simulink model "Main_Model"  (R2022b)
settings: Solver=VariableStepAuto  StartTime=0.0  StopTime=2  FixedStep=1e-4  RelTol=1e-6
InitFcn:
  | Lfg=1.75e-3;
  | Lfc=3.5e-3;
  | Lf = Lfg +Lfc;
  | Cf=20e-6;
  | 
  | Lg=0.0035;
  | L=Lf+Lg;
  | Rg=0.5498*2;
  | k=0.707;
  | omega0 = 100*pi;
  | kp1=10;
  | ki1=250;
  | %kp1=10;
  | %ki1=250;
  | kp2=10;
  | ki2=250;
undefined symbols (not defined in the file): den_Tn2p_11, den_Tn2p_12, den_Tp2n_11, den_Tp2n_12, num_Tn2p_11, num_Tn2p_12, num_Tp2n_11, num_Tp2n_12
libraries: spsSeriesRLCBranchLib x12, slpidlib x9, spsControlledVoltageSourceLib x6, spsThreePhaseVIMeasurementLib x3, spsAlphaBetaZerotoabcLib x2, simulink x2, spsGroundLib x1, spspowerguiLib x1
(part 1 of 2)
settings Model: Creator=Sweet_J  LastModifiedBy=Sweet_J
settings DataIOCC: ReturnWorkspaceOutputs=off

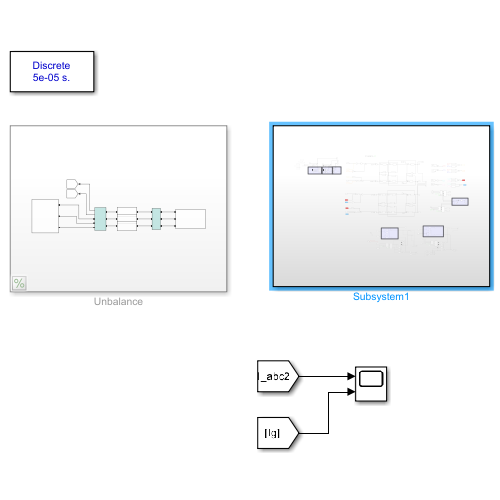
[thumbnail: Simulink's stored preview of the top-level diagram]
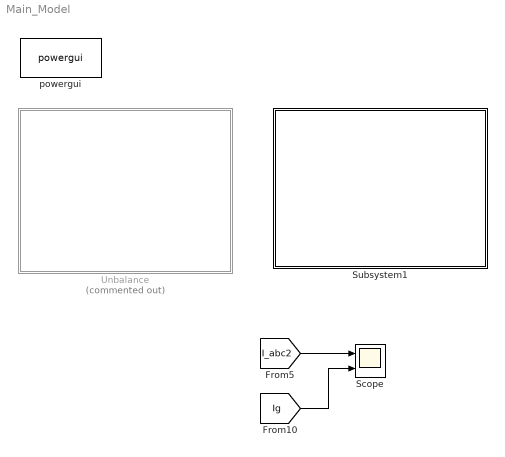
== system Main_Model ==
  Scope : Scope  NumInputPorts=2
  Subsystem1 : Subsystem
  Unbalance : Subsystem  Commented=on
  powergui : spspowerguiLib/powergui  Priority=1  SimulationMode=Discrete  SampleTime=5e-5  frequency=60  Iterations=50  frequencyindice=0  Pbase=100e6  ErrMax=1e-4  UnitsV=kV  UnitsW=MW  buscounter=0  FunctionMessages=off  echomessages=off  EnableUseOfTLC=off  CurrentSourceSwitches=off  DisableSnubberDevices=off  DisableRonSwitches=off  DisableVfSwitches=off  DisplayEquations=off  AutomaticDiscreteSolvers=off  SolverType=Tustin/Backward Euler (TBE)  Interpol=off  ExternalGateDelay=off  methode=off  Ts=100  x0status=blocks  SPID=on  SwTol=0  HookPort=off  NonlinearTolerance=1e-4  nMaxIteration=100  ContinueOnMaxIteration=off  RestoreLinks=warning  ResistiveCurrentMeasurement=off  Frange=[0:2:500]  Ylog=off  Xlog=on  ShowGrid=off  save=off  variable=ZData  structure=0  ZoomFFT=off  StartTime=0.0  cycles=1  DisplayStyle=1  fundamental=60  FreqAxis=off  MaxFrequency=1000  frequencyindicesteady=1  RmsSteady=1  display=off
  wires:
  [I_abc2] -> Scope/1
  [Ig] -> Scope/2

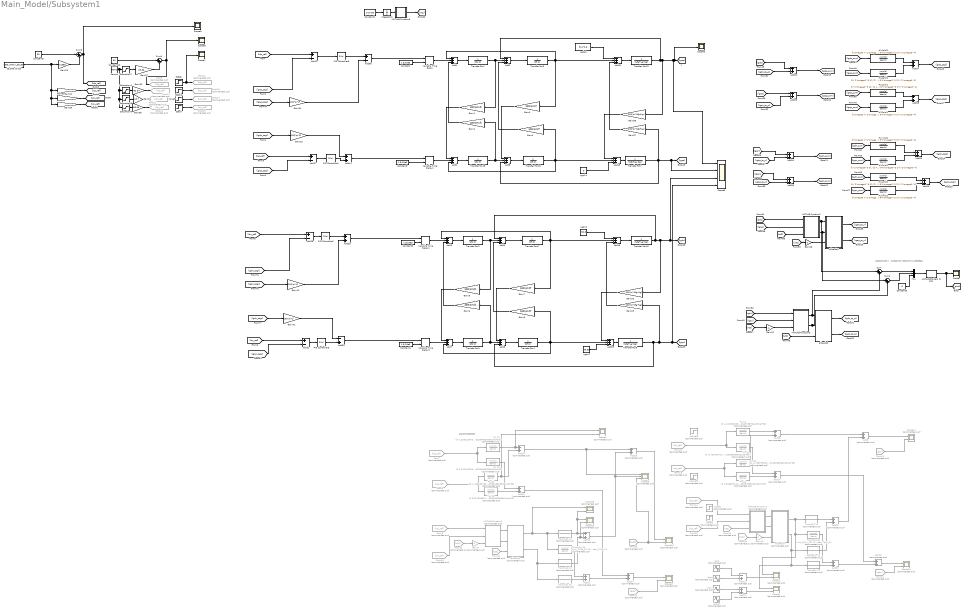
== system Main_Model/Subsystem1 ==
  note: 验证所求传函矩阵
  note: 这里其实说明了，系统真正的三相电流可以从哪里看出
  Add1 : Sum  Inputs=-++
  Add{9..10,12,14..15,17..18,20..23,25,27} (13 alike) : Sum  Commented=on
  Add11 : Sum  Commented=on  Inputs=-+
  Add2 : Sum  Inputs=-++
  Add24 : Sum  Inputs=-++
  Add{26,32..35,37..40,44} (10 alike) : Sum
  Add{28,31,36,42,47} (5 alike) : Sum  Inputs=+-
  Add29 : Sum  Inputs=++-
  Add{3..6,43,45} (6 alike) : Sum  Inputs=-+-
  Add30 : Sum  Inputs=-+
  Add7 : Sum  Inputs=++-
  Add8 : Sum  Inputs=++-
  Alpha-Beta-Zero to abc : spsAlphaBetaZerotoabcLib/Alpha-Beta-Zero to abc
      settings: LibrarySourceBlock=|
      | sps_lib/Control/Alpha-Beta-Zero
      | to abc
  Constant{,2..4} (4 alike) : Constant  Value=1.5/10e3
  Constant1 : Constant  Value=2*pi*50
  Constant10 : Constant  Value=50
  Constant5 : Constant  Value=0
  Constant9 : Constant  Value=50
  From10 : From  Commented=on  GotoTag=iqn_ref
  From{11..12,18..19} (4 alike) : From  Commented=on  GotoTag=wt2
  From13 : From  Commented=on  GotoTag=iqn_ref
  From14 : From  Commented=on  GotoTag=idp_ref
  From15 : From  Commented=on  GotoTag=iqp_ref
  From16 : From  Commented=on  GotoTag=igdp
  From17 : From  Commented=on  GotoTag=igqp
  From20 : From  Commented=on  GotoTag=igdn
  From21 : From  Commented=on  GotoTag=igqn
  From22 : From  Commented=on  GotoTag=idn_ref
  From7 : From  Commented=on  GotoTag=idp_ref
  From8 : From  Commented=on  GotoTag=iqp_ref
  From9 : From  Commented=on  GotoTag=idn_ref
  Gain{1..2,5..6} (4 alike) : Gain  Gain=100*pi*Lfc
  Gain10 : Gain  Commented=on  Gain=-1
  Gain22 : Gain  Gain=-1
  Gain{23,34,41..42} (4 alike) : Gain  Gain=100*pi*Lf
  Gain{25..26,37..38} (4 alike) : Gain  Gain=100*pi*(Lfg+Lg)
  Gain27 : Gain  Gain=25.56
  Gain28 : Gain  Gain=-1
  Gain29 : Gain  Gain=0.2556
  Gain{3..4,7..8} (4 alike) : Gain  Gain=100*pi*Cf
  Gain30 : Gain  Gain=-52.34
  Gain31 : Gain  Gain=-15.7
  Gain32 : Gain  Gain=-0.5234
  Gain33 : Gain  Gain=-0.157
  Gain35 : Gain  Gain=-0.5556
  Gain36 : Gain  Gain=-55.56
  Gain9 : Gain  Commented=on  Gain=-1
  Goto10 : Goto  Commented=on  GotoTag=iqp_ref
  Goto11 : Goto  Commented=on  GotoTag=idp_ref
  Goto12 : Goto  Commented=on  GotoTag=idn_ref
  Goto13 : Goto  Commented=on  GotoTag=iqp_ref
  Goto14 : Goto  Commented=on  GotoTag=idn_ref
  Goto15 : Goto  Commented=on  GotoTag=iqn_ref
  Goto16 : Goto  Commented=on  GotoTag=iqn_ref
  Goto9 : Goto  Commented=on  GotoTag=idp_ref
  H11n(s)2 : TransferFcn  Numerator=[k*omega0 k^2*omega0^2 4*k*omega0^3 2*k^2*omega0^4]  Denominator=[2 4*k*omega0 (2*k^2*omega0^2+8*omega0^2) 8*k*omega0^3 2*k^2*omega0^4]
  H11p(s)2 : TransferFcn  Numerator=[k*omega0 k^2*omega0^2 4*k*omega0^3 2*k^2*omega0^4]  Denominator=[2 4*k*omega0 (2*k^2*omega0^2+8*omega0^2) 8*k*omega0^3 2*k^2*omega0^4]
  H12n(s)2 : TransferFcn  Numerator=[k^2*omega0^3 0]  Denominator=[2 4*k*omega0 (2*k^2*omega0^2+8*omega0^2) 8*k*omega0^3 2*k^2*omega0^4]
  H12p(s)2 : TransferFcn  Numerator=[-k^2*omega0^3 0]  Denominator=[2 4*k*omega0 (2*k^2*omega0^2+8*omega0^2) 8*k*omega0^3 2*k^2*omega0^4]
  H21n(s)2 : TransferFcn  Numerator=[-k^2*omega0^3 0]  Denominator=[2 4*k*omega0 (2*k^2*omega0^2+8*omega0^2) 8*k*omega0^3 2*k^2*omega0^4]
  H21p(s)1 : TransferFcn  Numerator=[k^2*omega0^3 0]  Denominator=[2 4*k*omega0 (2*k^2*omega0^2+8*omega0^2) 8*k*omega0^3 2*k^2*omega0^4]
  H22n(s)2 : TransferFcn  Numerator=[k*omega0 k^2*omega0^2 4*k*omega0^3 2*k^2*omega0^4]  Denominator=[2 4*k*omega0 (2*k^2*omega0^2+8*omega0^2) 8*k*omega0^3 2*k^2*omega0^4]
  H22p(s)1 : TransferFcn  Numerator=[k*omega0 k^2*omega0^2 4*k*omega0^3 2*k^2*omega0^4]  Denominator=[2 4*k*omega0 (2*k^2*omega0^2+8*omega0^2) 8*k*omega0^3 2*k^2*omega0^4]
  Igdnref2 : Step  Commented=on  Time=0.5  After=-15.7  SampleTime=0
  Igqnref2 : Step  Commented=on  Time=0.5  After=-55.56  SampleTime=0
  Integrator1 : Integrator
  MATLAB Function1 : MATLAB Function  Commented=on  TreatAsAtomicUnit=on
  MATLAB Function2 : MATLAB Function  TreatAsAtomicUnit=on
  MATLAB Function3 : MATLAB Function  TreatAsAtomicUnit=on
  MATLAB Function4 : MATLAB Function  Commented=on  TreatAsAtomicUnit=on
  MATLAB Function5 : MATLAB Function  TreatAsAtomicUnit=on
  Mux : Mux  Inputs=3
  PID Controller{1..3,8} (4 alike) : slpidlib/PID Controller  Controller=PI  Form=Parallel  TimeDomain=Continuous-time  UseExternalTs=off  SampleTime=-1  IntegratorMethod=Forward Euler  FilterMethod=Forward Euler  ControllerParametersSource=internal  P=kp2  I=ki2  UseKiTs=off  D=0  N=100  UseFilter=on  TunerSelectOption=Transfer Function Based (PID Tuner App)  InitialConditionSource=internal  InitialConditionForIntegrator=0  InitialConditionForFilter=0  DifferentiatorICPrevScaledInput=0  ExternalReset=none  TrackingMode=off  Kt=1  LimitOutput=off  SatLimitsSource=internal  UpperSaturationLimit=5  LowerSaturationLimit=-5  LinearizeAsGain=on  AntiWindupMode=none  Kb=1  LimitIntegrator=off  UpperIntegratorSaturationLimit=inf  LowerIntegratorSaturationLimit=-inf  POutMin=[]  POutMax=[]  IOutMin=[]  IOutMax=[]  DOutMin=[]  DOutMax=[]  NOutMin=[]  NOutMax=[]  SumOutMin=[]  SumOutMax=[]  SaturationOutMin=[]  SaturationOutMax=[]  PParamMin=[]  PParamMax=[]  IParamMin=[]  IParamMax=[]  DParamMin=[]  DParamMax=[]  NParamMin=[]  NParamMax=[]  KbParamMin=[]  KbParamMax=[]  KtParamMin=[]  KtParamMax=[]  KbOutMin=[]  KbOutMax=[]  KtOutMin=[]  KtOutMax=[]  IntegratorOutMin=[]  IntegratorOutMax=[]  FilterOutMin=[]  FilterOutMax=[]  SumI1OutMin=[]  SumI1OutMax=[]  SumI2OutMin=[]  SumI2OutMax=[]  SumI3OutMin=[]  SumI3OutMax=[]  SumI4OutMin=[]  SumI4OutMax=[]  SumDOutMin=[]  SumDOutMax=[]  DifferentiatorOutMin=[]  DifferentiatorOutMax=[]  FilterDiffOutCoefMin=[]  FilterDiffOutCoefMax=[]  ReciprocalOutMin=[]  ReciprocalOutMax=[]  SumDenOutMin=[]  SumDenOutMax=[]  SumNumOutMin=[]  SumNumOutMax=[]  DivideOutMin=[]  DivideOutMax=[]  UdiffTsProdOutMin=[]  UdiffTsProdOutMax=[]  NTsProdOutMin=[]  NTsProdOutMax=[]  UintegralTsProdOutMin=[]  UintegralTsProdOutMax=[]  UngainTsProdOutMin=[]  UngainTsProdOutMax=[]  ClampingZeroOutDataTypeStr=Inherit: Inherit via back propagation  ClampingZeroOutMin=[]  ClampingZeroOutMax=[]  FilterDenConstantOutDataTypeStr=Inherit: Inherit via back propagation  FilterDenConstantOutMin=[]  FilterDenConstantOutMax=[]  PCopyOutDataTypeStr=Inherit: Inherit via back propagation  PCopyOutMin=[]  PCopyOutMax=[]  NCopyOutDataTypeStr=Inherit: Inherit via back propagation  NCopyOutMin=[]  NCopyOutMax=[]  IntegratorContinuousStateAttributes=''  IntegratorStateMustResolveToSignalObject=off  IntegratorRTWStateStorageClass=Auto  FilterContinuousStateAttributes=''  FilterStateMustResolveToSignalObject=off  FilterRTWStateStorageClass=Auto  ParallelPVariant=InternalParameters  IdealPVariant=Disabled  IVariant=InternalParameters  DVariant=Disabled  IntegratorVariant=Continuous  SatVariant=Disabled  AWVariant=Passthrough  PCopyVariant=Disabled  TRVariant=Disabled  FdbkBlocksVariant=Forward  IdealPFdbkVariant=Disabled  SatFdbkVariant=Disabled  DerivativeFilterVariant=Disabled  NVariant=Disabled  NCopyVariant=Disabled_SignalSpec  FilterICVariant=Disabled  IntegratorICVariant=InternalICs  ExternalResetVariant=Disabled  TRSumVariant=Passthrough  SumFdbkVariant=Disabled  SumVariant=Sum_PI  TsampFilterVariant=InternalTs  TsampNgainVariant=Passthrough  TsampIntegralVariant=Passthrough  ExternalSaturationOutDataTypeStr=Inherit: Same as second input
  Ramp4 : simulink/Sources/Ramp  slope=1/0.05  start=0.5  InitialOutput=0
  S5_500-优化值 : FromWorkspace  VariableName=data_matrix_S5_500  SampleTime=1e-4  OutputAfterFinalValue=Holding final value
  Saturation{4..7} (4 alike) : Saturate  UpperLimit=1
  Scope{,5..7,9} (5 alike) : Scope
  Scope{1..2,4,10..14,16} (9 alike) : Scope  Commented=on  NumInputPorts=2
  Scope3 : Scope  NumInputPorts=4
  Scope8 : Scope  Commented=on  NumInputPorts=3
  Step7 : Step  Time=0.5  After=-55.56  SampleTime=0
  Sum : Sum  Inputs=|++
  Sum1 : Sum  Inputs=|++
  Sum5 : Sum  Inputs=|+-
  Sum6 : Sum  Inputs=|+-
  Tn_11 : TransferFcn  Commented=on  Numerator="[0\t-1.01989600835735e-05\t-1.17900641885587\t27210822483.3065\t2.20664229038769e+15\t6.24118002886548e+19\t2.23888969085823e+23\t-1.87897168317480e+28\t-1.72747667412133e+31\t1.49299225089427e+37\t3.46754860086783e+41\t3.72395139767584e+45\t2.75969527472527e+49\t2.13218589100970e+53\t7.75699540504486e+56\t4.72648195947321e+60\t8.87634219530409e+63\t3.90830665381887e+67\t3.37200315132574e+70\t5.07472961316367e+73\t2.90981583243429e+76\t2.03203948734923e+79\t7.99056387196165e+81\t2.55933616110458e+84\t5.67621915091599e+86\t8.56295738691479e+88\t1.11882265410070e+91\t4.19269885253059e+92\t4.62854501341626e+93\t1.05501449453161e+90]"  Denominator="[1\t161278.621717248\t12035279516.7795\t542695985224921\t1.63257064864896e+19\t3.43390119397054e+23\t5.20049258153112e+27\t5.86772441336057e+31\t5.22760881524642e+35\t3.91267714232162e+39\t2.45413237239549e+43\t1.26235138927125e+47\t6.03726802536307e+50\t2.07018153285052e+54\t7.71850484834772e+57\t1.60031377689575e+61\t4.41534429030222e+64\t4.42330190486357e+67\t6.10017406906532e+70\t3.90204803066969e+73\t3.02442391656399e+76\t1.31463112199984e+79\t6.03213029135759e+81\t1.66887439356409e+84\t4.66750897142887e+86\t7.17549900075772e+88\t1.10373386868736e+91\t4.20898521075049e+92\t4.62821769543011e+93\t-2.01082889062291e+90]"
  Tn_12 : TransferFcn  Commented=on  Numerator="[0\t-4.73887980077529e-07\t-0.118436122586675\t-9193.30022294537\t-25646023787018.2\t-2.07793020544197e+18\t-5.82766629864322e+22\t-1.74505672449969e+26\t1.86276154721117e+31\t1.74470630730339e+34\t-1.43701084661191e+40\t-3.26090058003804e+44\t-3.26037804347025e+48\t-2.06927357042730e+52\t-1.50382199874050e+56\t-4.36162665974338e+59\t-2.45036259999236e+63\t-3.47377720397907e+66\t-1.31801840386399e+70\t-9.21889552517163e+72\t-1.38149069182804e+76\t-6.51712223024236e+78\t-4.53944031524944e+81\t-1.44387747033367e+84\t-3.90301534160538e+86\t-5.52809852598918e+88\t-2.66091379078351e+90\t-3.75543559155808e+91\t-1.49408154389136e+89\t-7.00886380960308e+89]"  Denominator="[1\t161278.621717248\t12035279516.7795\t542695985224921\t1.63257064864896e+19\t3.43390119397054e+23\t5.20049258153112e+27\t5.86772441336057e+31\t5.22760881524642e+35\t3.91267714232162e+39\t2.45413237239549e+43\t1.26235138927125e+47\t6.03726802536307e+50\t2.07018153285052e+54\t7.71850484834772e+57\t1.60031377689575e+61\t4.41534429030222e+64\t4.42330190486357e+67\t6.10017406906532e+70\t3.90204803066969e+73\t3.02442391656399e+76\t1.31463112199984e+79\t6.03213029135759e+81\t1.66887439356409e+84\t4.66750897142887e+86\t7.17549900075772e+88\t1.10373386868736e+91\t4.20898521075049e+92\t4.62821769543011e+93\t-2.01082889062291e+90]"
  Tn_21 : TransferFcn  Commented=on  Numerator="[0\t-2.72575672494487e-05\t-2.67780697081252\t-114599.451612093\t25642942591020.4\t2.07787868086678e+18\t5.82758566377686e+22\t1.74491674822968e+26\t-1.86277964459509e+31\t-1.74482881481782e+34\t1.43701045799572e+40\t3.26090034418790e+44\t3.26037826604666e+48\t2.06927358937222e+52\t1.50382192123535e+56\t4.36162780809189e+59\t2.45036177516416e+63\t3.47378233210236e+66\t1.31801708965542e+70\t9.21896059568848e+72\t1.38148936783182e+76\t6.51716065391267e+78\t4.53943833205246e+81\t1.44387765769510e+84\t3.90311991195425e+86\t5.52841692189602e+88\t2.66100296918848e+90\t3.75453399799371e+91\t-1.15709472803773e+89\t-4.22449198140034e+88]"  Denominator="[1\t161278.621717248\t12035279516.7795\t542695985224921\t1.63257064864896e+19\t3.43390119397054e+23\t5.20049258153112e+27\t5.86772441336057e+31\t5.22760881524642e+35\t3.91267714232162e+39\t2.45413237239549e+43\t1.26235138927125e+47\t6.03726802536307e+50\t2.07018153285052e+54\t7.71850484834772e+57\t1.60031377689575e+61\t4.41534429030222e+64\t4.42330190486357e+67\t6.10017406906532e+70\t3.90204803066969e+73\t3.02442391656399e+76\t1.31463112199984e+79\t6.03213029135759e+81\t1.66887439356409e+84\t4.66750897142887e+86\t7.17549900075772e+88\t1.10373386868736e+91\t4.20898521075049e+92\t4.62821769543011e+93\t-2.01082889062291e+90]"
  Tn_22 : TransferFcn  Commented=on  Numerator="[0\t3.66865324272166e-06\t-0.371826229889401\t27210820197.5691\t2.20664078258463e+15\t6.24117473554497e+19\t2.23888231391279e+23\t-1.87897185981957e+28\t-1.72747197520496e+31\t1.49299226921904e+37\t3.46754859641349e+41\t3.72395142079573e+45\t2.75969522576048e+49\t2.13218587839097e+53\t7.75699545713972e+56\t4.72648184009947e+60\t8.87634279451460e+63\t3.90830630184088e+67\t3.37200348967812e+70\t5.07472544820159e+73\t2.90981176456342e+76\t2.03203651448596e+79\t7.99054716401335e+81\t2.55934516074338e+84\t5.67629559985087e+86\t8.56289570963446e+88\t1.11878390677472e+91\t4.19253851985844e+92\t4.62825157508569e+93\t-2.00117520670361e+90]"  Denominator="[1\t161278.621717248\t12035279516.7795\t542695985224921\t1.63257064864896e+19\t3.43390119397054e+23\t5.20049258153112e+27\t5.86772441336057e+31\t5.22760881524642e+35\t3.91267714232162e+39\t2.45413237239549e+43\t1.26235138927125e+47\t6.03726802536307e+50\t2.07018153285052e+54\t7.71850484834772e+57\t1.60031377689575e+61\t4.41534429030222e+64\t4.42330190486357e+67\t6.10017406906532e+70\t3.90204803066969e+73\t3.02442391656399e+76\t1.31463112199984e+79\t6.03213029135759e+81\t1.66887439356409e+84\t4.66750897142887e+86\t7.17549900075772e+88\t1.10373386868736e+91\t4.20898521075049e+92\t4.62821769543011e+93\t-2.01082889062291e+90]"
  Tp_11 : TransferFcn  Commented=on  Numerator="[0\t-1.25322284335350e-05\t-2.02740537788495\t27210737835.9859\t2.20663793840066e+15\t6.24116626296036e+19\t2.23886077261772e+23\t-1.87897588898611e+28\t-1.72752135679541e+31\t1.49299184770071e+37\t3.46754821681792e+41\t3.72395106130426e+45\t2.75969508892492e+49\t2.13218578823217e+53\t7.75699430851545e+56\t4.72648172209308e+60\t8.87633831828796e+63\t3.90830600643315e+67\t3.37199825873036e+70\t5.07472177909344e+73\t2.90980757242417e+76\t2.03202861702974e+79\t7.99052798454746e+81\t2.55932291602922e+84\t5.67622759908534e+86\t8.56290284779787e+88\t1.11878404420830e+91\t4.19254404340210e+92\t4.62834852627690e+93]"  Denominator="[1\t161278.621529395\t12035279456.2977\t542695979191906\t1.63257061733538e+19\t3.43390109552110e+23\t5.20049238260333e+27\t5.86772414805569e+31\t5.22760856883647e+35\t3.91267695209602e+39\t2.45413222504702e+43\t1.26235129378665e+47\t6.03726748464878e+50\t2.07018118935140e+54\t7.71850362457027e+57\t1.60031311177394e+61\t4.41534276008939e+64\t4.42329659655974e+67\t6.10016546580316e+70\t3.90203985540913e+73\t3.02441198394233e+76\t1.31462548198536e+79\t6.03210232716645e+81\t1.66887043911015e+84\t4.66748787692584e+86\t7.17548130205310e+88\t1.10372137417744e+91\t4.20897950841205e+92\t4.62834862809614e+93]"
  Tp_12 : TransferFcn  Commented=on  Numerator="[0\t-1.18608236314470e-05\t-1.75109677806806\t-114697.716307309\t25641287601788.2\t2.07781430026798e+18\t5.82747088748898e+22\t1.74480497060541e+26\t-1.86278961312241e+31\t-1.74496642291660e+34\t1.43700919800844e+40\t3.26089973839346e+44\t3.26037735424563e+48\t2.06927349019002e+52\t1.50382186060258e+56\t4.36162596446295e+59\t2.45036239722728e+63\t3.47377484676323e+66\t1.31801807759520e+70\t9.21888581644634e+72\t1.38148983839453e+76\t6.51708864184348e+78\t4.53943011483970e+81\t1.44387260922491e+84\t3.90302852492583e+86\t5.52817130126409e+88\t2.66083943958935e+90\t3.75471287071865e+91\t-1.93887588410211e+87]"  Denominator="[1\t161278.621529395\t12035279456.2977\t542695979191906\t1.63257061733538e+19\t3.43390109552110e+23\t5.20049238260333e+27\t5.86772414805569e+31\t5.22760856883647e+35\t3.91267695209602e+39\t2.45413222504702e+43\t1.26235129378665e+47\t6.03726748464878e+50\t2.07018118935140e+54\t7.71850362457027e+57\t1.60031311177394e+61\t4.41534276008939e+64\t4.42329659655974e+67\t6.10016546580316e+70\t3.90203985540913e+73\t3.02441198394233e+76\t1.31462548198536e+79\t6.03210232716645e+81\t1.66887043911015e+84\t4.66748787692584e+86\t7.17548130205310e+88\t1.10372137417744e+91\t4.20897950841205e+92\t4.62834862809614e+93]"
  Tp_21 : TransferFcn  Commented=on  Numerator="[0\t2.94216760674153e-05\t4.42093407247836\t300641.920787539\t-25633527507541.4\t-2.07759953751829e+18\t-5.82705540457892e+22\t-1.74422205010133e+26\t1.86285087700518e+31\t1.74546015222327e+34\t-1.43700600599724e+40\t-3.26089770519802e+44\t-3.26037591493240e+48\t-2.06927290231164e+52\t-1.50382156142686e+56\t-4.36162560590497e+59\t-2.45036234473766e+63\t-3.47377754442195e+66\t-1.31801819198073e+70\t-9.21892944521939e+72\t-1.38148590156662e+76\t-6.51711111353095e+78\t-4.53942941502323e+81\t-1.44387357287478e+84\t-3.90304696099191e+86\t-5.52822127622576e+88\t-2.66087906457575e+90\t-3.75479198654529e+91\t3.61407592855685e+86]"  Denominator="[1\t161278.621529395\t12035279456.2977\t542695979191906\t1.63257061733538e+19\t3.43390109552110e+23\t5.20049238260333e+27\t5.86772414805569e+31\t5.22760856883647e+35\t3.91267695209602e+39\t2.45413222504702e+43\t1.26235129378665e+47\t6.03726748464878e+50\t2.07018118935140e+54\t7.71850362457027e+57\t1.60031311177394e+61\t4.41534276008939e+64\t4.42329659655974e+67\t6.10016546580316e+70\t3.90203985540913e+73\t3.02441198394233e+76\t1.31462548198536e+79\t6.03210232716645e+81\t1.66887043911015e+84\t4.66748787692584e+86\t7.17548130205310e+88\t1.10372137417744e+91\t4.20897950841205e+92\t4.62834862809614e+93]"
  Tp_22 : TransferFcn  Commented=on  Numerator="[0\t3.60780582170835e-06\t0.508903300575527\t27210914613.7454\t2.20664521469668e+15\t6.24118611598372e+19\t2.23889957097262e+23\t-1.87897006618828e+28\t-1.72745122527653e+31\t1.49299249961866e+37\t3.46754864365711e+41\t3.72395127329797e+45\t2.75969521169702e+49\t2.13218581722092e+53\t7.75699456142154e+56\t4.72648171699777e+60\t8.87633866859007e+63\t3.90830591483511e+67\t3.37199835513012e+70\t5.07472114504140e+73\t2.90980609802614e+76\t2.03203336431316e+79\t7.99052910989882e+81\t2.55933700246574e+84\t5.67627031006410e+86\t8.56293334609155e+88\t1.11878556056281e+91\t4.19254427849679e+92\t4.62834263680031e+93]"  Denominator="[1\t161278.621529395\t12035279456.2977\t542695979191906\t1.63257061733538e+19\t3.43390109552110e+23\t5.20049238260333e+27\t5.86772414805569e+31\t5.22760856883647e+35\t3.91267695209602e+39\t2.45413222504702e+43\t1.26235129378665e+47\t6.03726748464878e+50\t2.07018118935140e+54\t7.71850362457027e+57\t1.60031311177394e+61\t4.41534276008939e+64\t4.42329659655974e+67\t6.10016546580316e+70\t3.90203985540913e+73\t3.02441198394233e+76\t1.31462548198536e+79\t6.03210232716645e+81\t1.66887043911015e+84\t4.66748787692584e+86\t7.17548130205310e+88\t1.10372137417744e+91\t4.20897950841205e+92\t4.62834862809614e+93]"
  Transfer Fcn{1..3,18} (4 alike) : TransferFcn  Denominator=[Lfc 0]
  Transfer Fcn{7..8,13,16} (4 alike) : TransferFcn  Denominator=[(Lfg+Lg) Rg]
  Transfer Fcn{4..6,19} (4 alike) : TransferFcn  Denominator=[Cf 0]
  Tsumn2p_11 : TransferFcn  Commented=on  Numerator=num_Tn2p_11  Denominator=den_Tn2p_11
  Tsumn2p_12 : TransferFcn  Commented=on  Numerator=num_Tn2p_12  Denominator=den_Tn2p_12
  Tsumn2p_21 : TransferFcn  Commented=on  Numerator=num_Tn2p_12*(-1)  Denominator=den_Tn2p_12
  Tsumn2p_22 : TransferFcn  Commented=on  Numerator=num_Tn2p_11  Denominator=den_Tn2p_11
  Tsump2n_11 : TransferFcn  Commented=on  Numerator=num_Tp2n_11  Denominator=den_Tp2n_11
  Tsump2n_12 : TransferFcn  Commented=on  Numerator=num_Tp2n_12  Denominator=den_Tp2n_12
  Tsump2n_21 : TransferFcn  Commented=on  Numerator=num_Tp2n_12*(-1)  Denominator=den_Tp2n_11
  Tsump2n_22 : TransferFcn  Commented=on  Numerator=num_Tp2n_11  Denominator=den_Tp2n_11
  Variable Time Delay{,1..3} (4 alike) : VariableTransportDelay  MaximumDelay=10
  albe-dq1 : MATLAB Function  Commented=on  TreatAsAtomicUnit=on
  albe-dq2 : MATLAB Function  TreatAsAtomicUnit=on
  albe-dq3 : MATLAB Function  TreatAsAtomicUnit=on
  albe-dq4 : MATLAB Function  Commented=on  TreatAsAtomicUnit=on
  idcos : Sin  Commented=on  Amplitude=24.44  Frequency=2*2*50*pi  Phase=pi/2  SampleTime=0
  idnref : Step  Time=0.5  After=-15.7  SampleTime=0
  idpref1 : Step  Commented=on  Time=0.5  Before=50  After=24.44  SampleTime=0
  idsin1 : Sin  Commented=on  Amplitude=24.44  Frequency=2*2*50*pi  SampleTime=0
  iqcos1 : Sin  Commented=on  Amplitude=-52.34  Frequency=2*2*50*pi  Phase=pi/2  SampleTime=0
  iqpref1 : Step  Commented=on  Time=0.5  After=-52.34  SampleTime=0
  iqsin : Sin  Commented=on  Amplitude=-52.34  Frequency=2*2*50*pi  SampleTime=0
  ugdn2 : Constant  Value=80.8
  ugdp1 : Constant  Value=311*0.6
  ugq+4 : Constant  Value=0
  ugqn2 : Constant  Value=46.65
  转换后 : Step  Time=0.5  Before=50  After=24.44  SampleTime=0
  转换后2 : Step  Time=0.5  After=-52.34  SampleTime=0
  tag scope: I_abc2=global
  wires:
  [igqn] -> MATLAB Function3/2(uq)
  albe-dq2/1(vd) -> [igdn_to_p]
  [igdp] -> Add32/1
  Add33/1 -> [igqp_sum]
  [wt2] -> Gain22/1
  [igdn] -> MATLAB Function3/1(ud)
  [wt2] -> albe-dq2/3(ph)
  [wt2] -> Gain28/1
  Gain22/1 -> MATLAB Function3/3(ph)
  [igqp] -> Add33/1
  albe-dq3/2(vq) -> [igqp_to_n]
  albe-dq3/1(vd) -> [igdp_to_n]
  Integrator1/1 -> MATLAB Function5/1(u)
  [igqp_sum] -> H22p(s)1/1
  [igdn_to_p] -> Add32/2
  H11p(s)2/1 -> Add37/1
  [igdp] -> MATLAB Function2/1(ud)
  [wt2] -> MATLAB Function2/3(ph)
  MATLAB Function2/2(ub) -> Sum1/1, albe-dq3/2(vbeta)  "v_bn"
  [igqn_sum] -> H12n(s)2/1
  [igqp] -> MATLAB Function2/2(uq)
  MATLAB Function2/1(ua) -> albe-dq3/1(valpha), Sum/1  "v_an"
  Add34/1 -> [igdn_sum]
  Gain28/1 -> albe-dq3/3(ph)
  H22n(s)2/1 -> Add40/2
  [igqp_to_n] -> Add35/2
  [igqn] -> Add35/1
  [igdp_sum] -> H11p(s)2/1
  H12p(s)2/1 -> Add37/2
  Add37/1 -> [igdp_sogi]
  albe-dq2/2(vq) -> [igqn_to_p]
  [igdp_sum] -> H21p(s)1/1
  H22p(s)1/1 -> Add38/2
  H12n(s)2/1 -> Add39/2
  [igqn_sum] -> H22n(s)2/1
  Add40/1 -> [igqn_sogi]
  Add30/1 -> Variable Time Delay3/1  "usq"
  ugdn2/1 -> Add45/1
  [igdn_sogi] -> Gain41/1
  Add35/1 -> [igqn_sum]
  [igqn_sogi] -> Gain42/1
  [igqp_sogi] -> Add47/2
  Add43/1 -> Transfer Fcn7/1
  [igdp_sogi] -> Gain23/1
  Transfer Fcn7/1 -> Gain37/1, Add5/3, Scope3/2, [igqp]  "igq+"
  ugq+4/1 -> Add43/3
  Add42/1 -> PID Controller8/1
  Add29/1 -> Transfer Fcn8/1
  H11n(s)2/1 -> Add39/1
  ugdp1/1 -> Add24/1
  Add36/1 -> Variable Time Delay/1  "usd"
  H21n(s)2/1 -> Add40/1
  [igdn_sum] -> H11n(s)2/1
  [igqn_to_p] -> Add33/2
  Gain34/1 -> Add36/2
  [igdp_to_n] -> Add34/2
  Gain37/1 -> Add24/3
  [igdn] -> Add34/1
  Add24/1 -> Transfer Fcn13/1
  [igdp_sogi] -> Add42/2
  Add47/1 -> PID Controller1/1
  PID Controller3/1 -> Add30/2
  Gain23/1 -> Add44/1
  [igqp_sogi] -> Gain34/1
  PID Controller8/1 -> Add36/1
  MATLAB Function3/2(ub) -> Sum1/2, albe-dq2/2(vbeta)  "v_bn"
  H21p(s)1/1 -> Add38/1
  Add38/1 -> [igqp_sogi]
  PID Controller2/1 -> Add26/1
  MATLAB Function3/1(ua) -> Sum/2, albe-dq2/1(valpha)  "v_an"
  Add28/1 -> PID Controller2/1
  Gain42/1 -> Add26/2
  [igdn_sum] -> H21n(s)2/1
  ugqn2/1 -> Add29/3
  Gain26/1 -> Add29/1
  Add31/1 -> PID Controller3/1
  Add45/1 -> Transfer Fcn16/1
  Gain25/1 -> Add45/3
  Add32/1 -> [igdp_sum]
  Constant1/1 -> Integrator1/1
  Add44/1 -> Variable Time Delay1/1  "usq"
  PID Controller1/1 -> Add44/2
  Gain38/1 -> Add43/1
  [igdn_sogi] -> Add28/2
  Gain41/1 -> Add30/1
  [igqp_sum] -> H12p(s)2/1
  Transfer Fcn13/1 -> Add2/1, Gain38/1, Scope3/1, Scope6/1, [igdp]  "igd+"
  Add39/1 -> [igdn_sogi]
  Constant/1 -> Variable Time Delay/2
  Constant2/1 -> Variable Time Delay1/2
  Constant3/1 -> Variable Time Delay2/2
  Add26/1 -> Variable Time Delay2/1  "usq"
  Constant4/1 -> Variable Time Delay3/2
  Sum/1 -> Mux/1
  Sum1/1 -> Mux/2
  Constant5/1 -> Mux/3
  Mux/1 -> Alpha-Beta-Zero to abc/1
  Alpha-Beta-Zero to abc/1 -> [I_abc2], Scope/1
  MATLAB Function5/1(y) -> [wt2]
  Variable Time Delay/1 -> Add1/2
  Transfer Fcn1/1 -> Gain1/1, Add2/2  "i1d+"
  Add2/1 -> Transfer Fcn5/1
  Transfer Fcn5/1 -> Add24/2, Gain3/1, Add1/1  "vc+"
  Add1/1 -> Transfer Fcn1/1
  Gain1/1 -> Add4/1
  Gain2/1 -> Add1/3
  Add4/1 -> Transfer Fcn18/1
  Transfer Fcn19/1 -> Add4/3, Add43/2, Gain4/1  "vc+"
  Add5/1 -> Transfer Fcn19/1
  Transfer Fcn18/1 -> Gain2/1, Add5/2  "i1q+"
  Variable Time Delay1/1 -> Add4/2
  Gain3/1 -> Add5/1
  Gain4/1 -> Add2/3
  Gain8/1 -> Add6/3
  Gain7/1 -> Add8/1
  Transfer Fcn3/1 -> Add8/2, Gain6/1  "i1q-"
  Add8/1 -> Transfer Fcn4/1
  Transfer Fcn4/1 -> Add29/2, Gain8/1, Add7/3  "vc-"
  Add7/1 -> Transfer Fcn3/1
  Gain6/1 -> Add3/3
  Gain5/1 -> Add7/1
  Add3/1 -> Transfer Fcn2/1
  Transfer Fcn6/1 -> Gain7/1, Add45/2, Add3/1  "vc-"
  Add6/1 -> Transfer Fcn6/1
  Transfer Fcn2/1 -> Add6/2, Gain5/1  "i1d-"
  Transfer Fcn16/1 -> Add6/1, Gain26/1, Scope3/3, [igdn]  "igd-"
  Transfer Fcn8/1 -> Scope3/4, [igqn], Gain25/1, Add8/3  "igq-"
  Variable Time Delay2/1 -> Add3/2
  Variable Time Delay3/1 -> Add7/2
  [igqn_sogi] -> Add31/2
  From7/1 -> Tp_11/1, Tp_21/1
  From22/1 -> Tn_11/1, Tn_21/1
  Tn_11/1 -> Add18/1
  Tn_21/1 -> Add17/1
  Gain9/1 -> MATLAB Function1/3(ph)
  MATLAB Function1/2(ub) -> albe-dq1/2(vbeta)  "v_bn"
  From12/1 -> Gain9/1
  From11/1 -> albe-dq1/3(ph)
  MATLAB Function1/1(ua) -> albe-dq1/1(valpha)  "v_an"
  From9/1 -> MATLAB Function1/1(ud)
  From10/1 -> MATLAB Function1/2(uq)
  From13/1 -> Tn_12/1, Tn_22/1
  Tn_22/1 -> Add17/2
  Tn_12/1 -> Add18/2
  Add18/1 -> Add9/1
  albe-dq1/2(vq) -> Tsumn2p_22/1, Tsumn2p_12/1
  Tsumn2p_11/1 -> Scope14/1, Scope16/2, Add20/1
  Tsumn2p_12/1 -> Scope14/2, Add20/2
  Tsumn2p_22/1 -> Add21/2
  Tsumn2p_21/1 -> Add21/1
  Add25/1 -> Scope10/1  "idp_theory"
  From16/1 -> Scope8/3, Scope10/2  "idp_simulation"
  Add27/1 -> Scope11/1  "iqp_theory"
  From17/1 -> Scope11/2  "iqp_simulation"
  Tsump2n_21/1 -> Add23/1
  Tsump2n_22/1 -> Add23/2
  Tsump2n_12/1 -> Add22/2
  Tsump2n_11/1 -> Add22/1
  From18/1 -> Gain10/1
  MATLAB Function4/2(ub) -> albe-dq4/2(vbeta)  "v_bn"
  MATLAB Function4/1(ua) -> albe-dq4/1(valpha)  "v_an"
  albe-dq4/1(vd) -> Tsump2n_11/1, Scope1/1, Tsump2n_21/1
  albe-dq4/2(vq) -> Scope2/1, Tsump2n_22/1, Tsump2n_12/1
  Add22/1 -> Add9/2
  From20/1 -> Scope12/2  "idn_simulation"
  Add23/1 -> Add10/2
  From21/1 -> Scope13/2  "iqn_simulation"
  From8/1 -> Tp_12/1, Tp_22/1
  Tp_11/1 -> Scope4/1, Add14/1
  Tp_21/1 -> Add15/1
  Tp_22/1 -> Add15/2
  Add14/1 -> Scope8/1, Add25/1
  Add15/1 -> Add27/1
  Add20/1 -> Add25/2, Scope8/2
  Add21/1 -> Add27/2
  Add17/1 -> Add10/1
  Add10/1 -> Scope13/1  "iqn_theory"
  Add9/1 -> Scope12/1  "idn_theory"
  iqsin/1 -> Add11/1
  idcos/1 -> Add11/2
  iqcos1/1 -> Add12/2
  idsin1/1 -> Add12/1
  Add11/1 -> Scope1/2  "d"
  Add12/1 -> Scope2/2  "q"
  From14/1 -> MATLAB Function4/1(ud)
  From15/1 -> MATLAB Function4/2(uq)
  From19/1 -> MATLAB Function4/3(ph)
  Gain10/1 -> albe-dq4/3(ph)
  [idp_ref] -> Add42/1
  [iqp_ref] -> Add47/1
  [idn_ref] -> Add28/1
  [iqn_ref] -> Add31/1
  albe-dq1/1(vd) -> Scope16/1, Tsumn2p_11/1, Tsumn2p_21/1
  Gain31/1 -> Goto12/1  "idn_ref"
  Saturation4/1 -> Gain30/1  "斜坡"
  Constant9/1 -> Sum5/1
  Gain29/1 -> Sum5/2  "优化idp_ref"
  Gain30/1 -> Goto10/1
  Saturation5/1 -> Gain31/1
  Sum6/1 -> Scope5/1, Goto9/1
  Gain27/1 -> Sum6/2
  Ramp4/1 -> Saturation4/1, Saturation6/1, Saturation5/1, Saturation7/1
  Constant10/1 -> Sum6/1
  Gain32/1 -> [iqp_ref]  "iqp_ref"
  Gain33/1 -> [idn_ref]  "idn_ref"
  Sum5/1 -> [idp_ref], Scope9/1  "idp_ref"
  Gain36/1 -> Goto16/1
  Saturation7/1 -> Gain27/1  "斜坡"
  Gain35/1 -> [iqn_ref]  "iqn_ref"
  Saturation6/1 -> Gain36/1
  Step7/1 -> Goto15/1
  idnref/1 -> Goto14/1
  转换后2/1 -> Goto13/1
  转换后/1 -> Scope7/1, Goto11/1
  Tp_12/1 -> Scope4/2, Add14/2
  S5_500-优化值/1 -> Gain32/1, Gain35/1, Gain33/1, Gain29/1

== system Main_Model/Unbalance ==
  Bus 0 : spsThreePhaseVIMeasurementLib/Three-Phase V-I Measurement  VoltageMeasurement=phase-to-ground  SetLabelV=off  LabelV=Vabc  Vpu=off  VpuLL=off  CurrentMeasurement=yes  SetLabelI=off  LabelI=Iabc  Ipu=off  Pbase=100e6  Vbase=500e3  OutputType=Complex  PhasorSimulation=off  PSBequivalent=0
  Bus 1 : spsThreePhaseVIMeasurementLib/Three-Phase V-I Measurement  VoltageMeasurement=phase-to-ground  SetLabelV=on  LabelV=V1  Vpu=off  VpuLL=off  CurrentMeasurement=no  SetLabelI=off  LabelI=I1  Ipu=off  Pbase=100e6  Vbase=500e3  OutputType=Complex  PhasorSimulation=off  PSBequivalent=0
  Grid : Subsystem
  IBR1 : Subsystem
  Series RLC Branch3 : spsSeriesRLCBranchLib/Series RLC Branch  LConnTagsString=__new0  RConnTagsString=__new0  BranchType=RL  Resistance=Rg  Inductance=Lg  SetiL0=off  InitialCurrent=0  Capacitance=1e-6  Setx0=off  InitialVoltage=0  Measurements=None
  Series RLC Branch4 : spsSeriesRLCBranchLib/Series RLC Branch  LConnTagsString=__new0  RConnTagsString=__new0  BranchType=RL  Resistance=Rg  Inductance=Lg  SetiL0=off  InitialCurrent=0  Capacitance=1e-6  Setx0=off  InitialVoltage=0  Measurements=None
  z1 : spsSeriesRLCBranchLib/Series RLC Branch  LConnTagsString=__new0  RConnTagsString=__new0  BranchType=RL  Resistance=Rg  Inductance=Lg  SetiL0=off  InitialCurrent=0  Capacitance=1e-6  Setx0=off  InitialVoltage=0  Measurements=None
  tag scope: Igabc=global, Vgabc=global
  wires:
  Bus 0/1 -> [Vgabc]
  Bus 0/2 -> [Igabc]
  connections:
  IBR1/RConn1 -- Bus 1/LConn1
  Grid/RConn1 -- Bus 0/RConn1
  IBR1/RConn3 -- Bus 1/LConn3
  IBR1/RConn2 -- Bus 1/LConn2
  Series RLC Branch3/LConn1 -- Bus 0/LConn1
  Grid/RConn2 -- Bus 0/RConn2
  Grid/RConn3 -- Bus 0/RConn3
  Bus 0/LConn2 -- Series RLC Branch4/LConn1
  Bus 0/LConn3 -- z1/LConn1
  Bus 1/RConn1 -- Series RLC Branch3/RConn1
  Series RLC Branch4/RConn1 -- Bus 1/RConn2
  z1/RConn1 -- Bus 1/RConn3

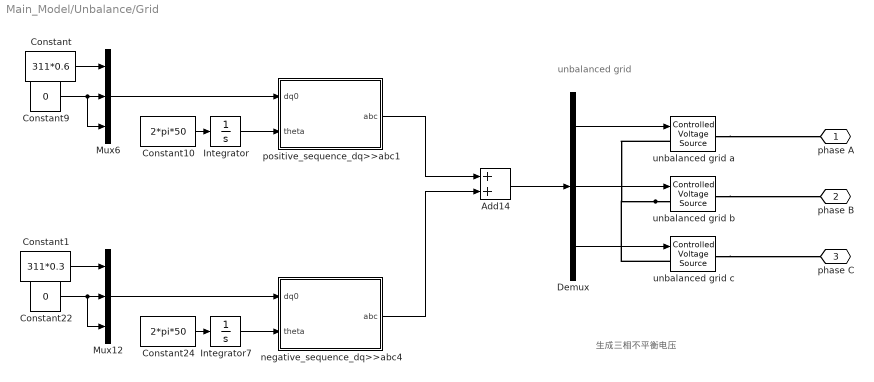
== system Main_Model/Unbalance/Grid ==
  note: unbalanced grid
  note: 生成三相不平衡电压
  Add14 : Sum
  Constant : Constant  Value=311*0.6
  Constant1 : Constant  Value=311*0.3
  Constant10 : Constant  Value=2*pi*50
  Constant22 : Constant  Value=0
  Constant24 : Constant  Value=2*pi*50
  Constant9 : Constant  Value=0
  Demux : Demux  Outputs=3
  Integrator : Integrator
  Integrator7 : Integrator  InitialCondition=-pi/6
  Mux12 : Mux  Inputs=3
  Mux6 : Mux  Inputs=3
  negative_sequence_dq>>abc4 : Subsystem
  positive_sequence_dq>>abc1 : Subsystem
  unbalanced grid a : spsControlledVoltageSourceLib/Controlled Voltage Source  Initialize=on  Source_Type=AC  Amplitude=0  Phase=0  Frequency=0  Measurements=None
  "unbalanced grid b " : spsControlledVoltageSourceLib/Controlled Voltage Source  Initialize=on  Source_Type=AC  Amplitude=0  Phase=0  Frequency=0  Measurements=None
  unbalanced grid c : spsControlledVoltageSourceLib/Controlled Voltage Source  Initialize=on  Source_Type=AC  Amplitude=0  Phase=0  Frequency=0  Measurements=None
  phase A : PMIOPort  Side=Right
  phase B : PMIOPort  Port=2  Side=Right
  phase C : PMIOPort  Port=3  Side=Right
  wires:
  negative_sequence_dq>>abc4/1(abc) -> Add14/2
  Mux12/1 -> negative_sequence_dq>>abc4/1(dq0)
  Integrator/1 -> positive_sequence_dq>>abc1/2(theta)
  Demux/2 -> "unbalanced grid b "/1
  Constant24/1 -> Integrator7/1
  positive_sequence_dq>>abc1/1(abc) -> Add14/1
  Constant9/1 -> Mux6/3, Mux6/2
  Mux6/1 -> positive_sequence_dq>>abc1/1(dq0)
  Constant10/1 -> Integrator/1
  Demux/3 -> unbalanced grid c/1
  Demux/1 -> unbalanced grid a/1
  Integrator7/1 -> negative_sequence_dq>>abc4/2(theta)
  Add14/1 -> Demux/1
  Constant22/1 -> Mux12/3, Mux12/2
  Constant/1 -> Mux6/1
  Constant1/1 -> Mux12/1
  connections:
  unbalanced grid c/RConn1 -- phase C/RConn1
  "unbalanced grid b "/LConn1 -- unbalanced grid a/LConn1 -- unbalanced grid c/LConn1
  "unbalanced grid b "/RConn1 -- phase B/RConn1
  unbalanced grid a/RConn1 -- phase A/RConn1

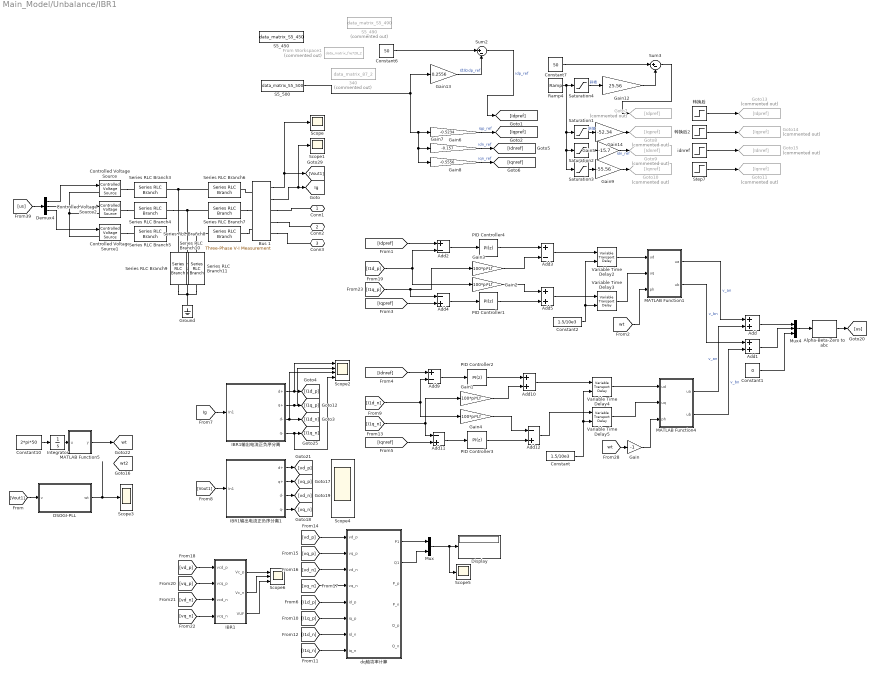
== system Main_Model/Unbalance/IBR1 ==
  340 : FromWorkspace  Commented=on  VariableName=data_matrix_87_2  SampleTime=1e-4  OutputAfterFinalValue=Holding final value
  Add{,1,5,10} (4 alike) : Sum
  Add11 : Sum  Inputs=-+
  Add12 : Sum  Inputs=-+
  Add2 : Sum  Inputs=+-
  Add3 : Sum  Inputs=+-
  Add4 : Sum  Inputs=-+
  Add9 : Sum  Inputs=+-
  Alpha-Beta-Zero to abc : spsAlphaBetaZerotoabcLib/Alpha-Beta-Zero to abc
      settings: LibrarySourceBlock=|
      | sps_lib/Control/Alpha-Beta-Zero
      | to abc
  Bus 1 : spsThreePhaseVIMeasurementLib/Three-Phase V-I Measurement  VoltageMeasurement=phase-to-ground  SetLabelV=off  LabelV=Vabc  Vpu=off  VpuLL=off  CurrentMeasurement=yes  SetLabelI=off  LabelI=Iabc  Ipu=off  Pbase=100e6  Vbase=500e3  OutputType=Complex  PhasorSimulation=off  PSBequivalent=0
  Constant : Constant  Value=1.5/10e3
  Constant1 : Constant  Value=0
  Constant10 : Constant  Value=2*pi*50
  Constant2 : Constant  Value=1.5/10e3
  Constant6 : Constant  Value=50
  Constant7 : Constant  Value=50
  Controlled Voltage Source : spsControlledVoltageSourceLib/Controlled Voltage Source  Initialize=on  Source_Type=AC  Amplitude=0  Phase=0  Frequency=0  Measurements=None
  Controlled Voltage Source1 : spsControlledVoltageSourceLib/Controlled Voltage Source  Initialize=on  Source_Type=AC  Amplitude=0  Phase=0  Frequency=0  Measurements=None
  Controlled Voltage Source2 : spsControlledVoltageSourceLib/Controlled Voltage Source  Initialize=on  Source_Type=AC  Amplitude=0  Phase=0  Frequency=0  Measurements=None
  DSOGI-PLL : Subsystem
  Demux4 : Demux  Outputs=3
  Display : Display
  From Workspace1 : FromWorkspace  Commented=on  VariableName=data_matrix_fre728_2  SampleTime=1e-4  OutputAfterFinalValue=Holding final value
  Gain : Gain  Gain=-1
  Gain{1..4} (4 alike) : Gain  Gain=100*pi*Lf
  Gain12 : Gain  Gain=25.56
  Gain13 : Gain  Gain=0.2556
  Gain14 : Gain  Gain=-52.34
  Gain5 : Gain  Gain=-15.7
  Gain6 : Gain  Gain=-0.5234
  Gain7 : Gain  Gain=-0.157
  Gain8 : Gain  Gain=-0.5556
  Gain9 : Gain  Gain=-55.56
  Goto10 : Goto  Commented=on  GotoTag=Iqnref
  Goto11 : Goto  Commented=on  GotoTag=Iqnref
  Goto13 : Goto  Commented=on  GotoTag=Idpref
  Goto14 : Goto  Commented=on  GotoTag=Iqpref
  Goto15 : Goto  Commented=on  GotoTag=Idnref
  Goto7 : Goto  Commented=on  GotoTag=Idpref
  Goto8 : Goto  Commented=on  GotoTag=Iqpref
  Goto9 : Goto  Commented=on  GotoTag=Idnref
  Ground : spsGroundLib/Ground  LConnTagsString=a
  IBR1 : MATLAB Function  TreatAsAtomicUnit=on
  IBR1输出电流正负序分离 : Subsystem
  IBR1输出电流正负序分离1 : Subsystem
  Integrator : Integrator
  MATLAB Function1 : MATLAB Function  TreatAsAtomicUnit=on
  MATLAB Function4 : MATLAB Function  TreatAsAtomicUnit=on
  MATLAB Function5 : MATLAB Function  TreatAsAtomicUnit=on
  Mux : Mux  Inputs=2
  Mux4 : Mux  Inputs=3
  PID Controller{1..4} (4 alike) : slpidlib/PID Controller  Controller=PI  Form=Parallel  TimeDomain=Discrete-time  UseExternalTs=off  SampleTime=-1  IntegratorMethod=Forward Euler  FilterMethod=Forward Euler  ControllerParametersSource=internal  P=kp1  I=ki1  UseKiTs=off  D=0  N=100  UseFilter=on  TunerSelectOption=Transfer Function Based (PID Tuner App)  InitialConditionSource=internal  InitialConditionForIntegrator=0  InitialConditionForFilter=0  DifferentiatorICPrevScaledInput=0  ExternalReset=none  TrackingMode=off  Kt=1  LimitOutput=off  SatLimitsSource=internal  UpperSaturationLimit=5  LowerSaturationLimit=-5  LinearizeAsGain=on  AntiWindupMode=none  Kb=1  LimitIntegrator=off  UpperIntegratorSaturationLimit=inf  LowerIntegratorSaturationLimit=-inf  POutMin=[]  POutMax=[]  IOutMin=[]  IOutMax=[]  DOutMin=[]  DOutMax=[]  NOutMin=[]  NOutMax=[]  SumOutMin=[]  SumOutMax=[]  SaturationOutMin=[]  SaturationOutMax=[]  PParamMin=[]  PParamMax=[]  IParamMin=[]  IParamMax=[]  DParamMin=[]  DParamMax=[]  NParamMin=[]  NParamMax=[]  KbParamMin=[]  KbParamMax=[]  KtParamMin=[]  KtParamMax=[]  KbOutMin=[]  KbOutMax=[]  KtOutMin=[]  KtOutMax=[]  IntegratorOutMin=[]  IntegratorOutMax=[]  FilterOutMin=[]  FilterOutMax=[]  SumI1OutMin=[]  SumI1OutMax=[]  SumI2OutMin=[]  SumI2OutMax=[]  SumI3OutMin=[]  SumI3OutMax=[]  SumI4OutMin=[]  SumI4OutMax=[]  SumDOutMin=[]  SumDOutMax=[]  DifferentiatorOutMin=[]  DifferentiatorOutMax=[]  FilterDiffOutCoefMin=[]  FilterDiffOutCoefMax=[]  ReciprocalOutMin=[]  ReciprocalOutMax=[]  SumDenOutMin=[]  SumDenOutMax=[]  SumNumOutMin=[]  SumNumOutMax=[]  DivideOutMin=[]  DivideOutMax=[]  UdiffTsProdOutMin=[]  UdiffTsProdOutMax=[]  NTsProdOutMin=[]  NTsProdOutMax=[]  UintegralTsProdOutMin=[]  UintegralTsProdOutMax=[]  UngainTsProdOutMin=[]  UngainTsProdOutMax=[]  ClampingZeroOutDataTypeStr=Inherit: Inherit via back propagation  ClampingZeroOutMin=[]  ClampingZeroOutMax=[]  FilterDenConstantOutDataTypeStr=Inherit: Inherit via back propagation  FilterDenConstantOutMin=[]  FilterDenConstantOutMax=[]  PCopyOutDataTypeStr=Inherit: Inherit via back propagation  PCopyOutMin=[]  PCopyOutMax=[]  NCopyOutDataTypeStr=Inherit: Inherit via back propagation  NCopyOutMin=[]  NCopyOutMax=[]  IntegratorContinuousStateAttributes=''  IntegratorStateMustResolveToSignalObject=off  IntegratorRTWStateStorageClass=Auto  FilterContinuousStateAttributes=''  FilterStateMustResolveToSignalObject=off  FilterRTWStateStorageClass=Auto  ParallelPVariant=InternalParameters  IdealPVariant=Disabled  IVariant=InternalParameters  DVariant=Disabled  IntegratorVariant=Discrete  SatVariant=Disabled  AWVariant=Passthrough  PCopyVariant=Disabled  TRVariant=Disabled  FdbkBlocksVariant=Forward  IdealPFdbkVariant=Disabled  SatFdbkVariant=Disabled  DerivativeFilterVariant=Disabled  NVariant=Disabled  NCopyVariant=Disabled_SignalSpec  FilterICVariant=Disabled  IntegratorICVariant=InternalICs  ExternalResetVariant=Disabled  TRSumVariant=Passthrough  SumFdbkVariant=Disabled  SumVariant=Sum_PI  TsampFilterVariant=InternalTs  TsampNgainVariant=Passthrough  TsampIntegralVariant=Passthrough  ExternalSaturationOutDataTypeStr=Inherit: Same as second input
  Ramp4 : simulink/Sources/Ramp  slope=1/0.05  start=0.5  InitialOutput=0
  S5_450 : FromWorkspace  VariableName=data_matrix_S5_450  SampleTime=1e-4  OutputAfterFinalValue=Holding final value
  S5_490 : FromWorkspace  Commented=on  VariableName=data_matrix_S5_490  SampleTime=1e-4  OutputAfterFinalValue=Holding final value
  S5_500 : FromWorkspace  VariableName=data_matrix_S5_500  SampleTime=1e-4  OutputAfterFinalValue=Holding final value
  Saturation{1..4} (4 alike) : Saturate  UpperLimit=1
  Scope{,1,3,5} (4 alike) : Scope
  Scope2 : Scope  NumInputPorts=4
  Scope4 : Scope  NumInputPorts=4
  Scope6 : Scope  NumInputPorts=3
  Series RLC Branch10 : spsSeriesRLCBranchLib/Series RLC Branch  LConnTagsString=__new0  RConnTagsString=__new0  BranchType=C  Resistance=1  Inductance=Lfg  SetiL0=off  InitialCurrent=0  Capacitance=Cf  Setx0=off  InitialVoltage=0  Measurements=None
  Series RLC Branch11 : spsSeriesRLCBranchLib/Series RLC Branch  LConnTagsString=__new0  RConnTagsString=__new0  BranchType=C  Resistance=1  Inductance=Lfg  SetiL0=off  InitialCurrent=0  Capacitance=Cf  Setx0=off  InitialVoltage=0  Measurements=None
  Series RLC Branch3 : spsSeriesRLCBranchLib/Series RLC Branch  LConnTagsString=__new0  RConnTagsString=__new0  BranchType=L  Resistance=1  Inductance=Lfc  SetiL0=off  InitialCurrent=0  Capacitance=1e-6  Setx0=off  InitialVoltage=0  Measurements=None
  Series RLC Branch4 : spsSeriesRLCBranchLib/Series RLC Branch  LConnTagsString=__new0  RConnTagsString=__new0  BranchType=L  Resistance=1  Inductance=Lfc  SetiL0=off  InitialCurrent=0  Capacitance=1e-6  Setx0=off  InitialVoltage=0  Measurements=None
  Series RLC Branch5 : spsSeriesRLCBranchLib/Series RLC Branch  LConnTagsString=__new0  RConnTagsString=__new0  BranchType=L  Resistance=1  Inductance=Lfc  SetiL0=off  InitialCurrent=0  Capacitance=1e-6  Setx0=off  InitialVoltage=0  Measurements=None
  Series RLC Branch6 : spsSeriesRLCBranchLib/Series RLC Branch  LConnTagsString=__new0  RConnTagsString=__new0  BranchType=L  Resistance=1  Inductance=Lfg  SetiL0=off  InitialCurrent=0  Capacitance=1e-6  Setx0=off  InitialVoltage=0  Measurements=None
  Series RLC Branch7 : spsSeriesRLCBranchLib/Series RLC Branch  LConnTagsString=__new0  RConnTagsString=__new0  BranchType=L  Resistance=1  Inductance=Lfg  SetiL0=off  InitialCurrent=0  Capacitance=1e-6  Setx0=off  InitialVoltage=0  Measurements=None
  Series RLC Branch8 : spsSeriesRLCBranchLib/Series RLC Branch  LConnTagsString=__new0  RConnTagsString=__new0  BranchType=L  Resistance=1  Inductance=Lfg  SetiL0=off  InitialCurrent=0  Capacitance=1e-6  Setx0=off  InitialVoltage=0  Measurements=None
  Series RLC Branch9 : spsSeriesRLCBranchLib/Series RLC Branch  LConnTagsString=__new0  RConnTagsString=__new0  BranchType=C  Resistance=1  Inductance=Lfg  SetiL0=off  InitialCurrent=0  Capacitance=Cf  Setx0=off  InitialVoltage=0  Measurements=None
  Step7 : Step  Time=0.5  After=-55.56  SampleTime=0
  Sum2 : Sum  Inputs=|+-
  Sum3 : Sum  Inputs=|+-
  Variable Time Delay{2..5} (4 alike) : VariableTransportDelay  MaximumDelay=10
  dq轴功率计算 : MATLAB Function  TreatAsAtomicUnit=on
  idnref : Step  Time=0.5  After=-15.7  SampleTime=0
  转换后 : Step  Time=0.5  Before=50  After=24.44  SampleTime=0
  转换后2 : Step  Time=0.5  After=-52.34  SampleTime=0
  Conn1 : PMIOPort  Side=Right
  Conn2 : PMIOPort  Port=2  Side=Right
  Conn3 : PMIOPort  Port=3  Side=Right
  tag scope: Ig=global, wt2=global, wt=global
  wires:
  Bus 1/1 -> Scope/1, [Vout1]
  Bus 1/2 -> Scope1/1, [Ig]
  IBR1输出电流正负序分离/2(q+) -> Scope2/2, [I1q_p]
  IBR1输出电流正负序分离/4(q-) -> Scope2/4, [I1q_n]
  [Ig] -> IBR1输出电流正负序分离/1(In1)
  PID Controller3/1 -> Add12/2
  PID Controller2/1 -> Add10/1
  Gain4/1 -> Add12/1
  Add9/1 -> PID Controller2/1
  MATLAB Function4/2(ub) -> Add1/2  "v_bn"
  Add2/1 -> PID Controller4/1
  Add11/1 -> PID Controller3/1
  Add4/1 -> PID Controller1/1
  Gain3/1 -> Add3/2
  PID Controller4/1 -> Add3/1
  Gain2/1 -> Add5/1
  Gain1/1 -> Add10/2
  PID Controller1/1 -> Add5/2
  [I1d_n] -> Gain4/1, Add9/2
  [I1q_n] -> Gain1/1, Add11/1
  MATLAB Function4/1(ua) -> Add/2  "v_an"
  [wt] -> Gain/1
  Demux4/3 -> Controlled Voltage Source1/1
  [us] -> Demux4/1
  Demux4/1 -> Controlled Voltage Source/1
  Demux4/2 -> Controlled Voltage Source2/1
  IBR1输出电流正负序分离/3(d-) -> [I1d_n], Scope2/3
  idnref/1 -> Goto15/1
  Step7/1 -> Goto11/1
  Mux4/1 -> Alpha-Beta-Zero to abc/1
  Constant1/1 -> Mux4/3
  Add10/1 -> Variable Time Delay4/1
  Gain/1 -> MATLAB Function4/3(ph)
  Add12/1 -> Variable Time Delay5/1
  Add5/1 -> Variable Time Delay3/1
  Add3/1 -> Variable Time Delay2/1
  [I1d_p] -> Gain2/1, Add2/2
  [I1q_p] -> Add4/1, Gain3/1
  [wt] -> MATLAB Function1/3(ph)
  MATLAB Function1/1(ua) -> Add/1  "v_an"
  MATLAB Function1/2(ub) -> Add1/1  "v_bn"
  Alpha-Beta-Zero to abc/1 -> [us]
  Constant/1 -> Variable Time Delay4/2, Variable Time Delay5/2
  Add/1 -> Mux4/1
  Add1/1 -> Mux4/2
  转换后2/1 -> Goto14/1
  转换后/1 -> Goto13/1
  IBR1输出电流正负序分离/1(d+) -> Scope2/1, [I1d_p]
  Variable Time Delay4/1 -> MATLAB Function4/1(ud)
  Variable Time Delay5/1 -> MATLAB Function4/2(uq)
  Variable Time Delay3/1 -> MATLAB Function1/2(uq)
  Constant2/1 -> Variable Time Delay2/2, Variable Time Delay3/2
  Variable Time Delay2/1 -> MATLAB Function1/1(ud)
  S5_500/1 -> Gain13/1, Gain6/1, Gain8/1, Gain7/1
  Integrator/1 -> MATLAB Function5/1(u)
  Constant10/1 -> Integrator/1
  [Vout1] -> DSOGI-PLL/1(v)
  Sum3/1 -> Goto7/1
  Saturation2/1 -> Gain5/1
  Gain9/1 -> Goto10/1
  Gain6/1 -> [Iqpref]  "iqp_ref"
  Gain8/1 -> [Iqnref]  "iqn_ref"
  Gain7/1 -> [Idnref]  "idn_ref"
  Sum2/1 -> [Idpref]  "idp_ref"
  [Idpref] -> Add2/1
  [Iqpref] -> Add4/2
  [Iqnref] -> Add11/2
  [Idnref] -> Add9/1
  [Vout1] -> IBR1输出电流正负序分离1/1(In1)
  DSOGI-PLL/1(wt) -> Scope3/1
  Constant6/1 -> Sum2/1
  Gain13/1 -> Sum2/2  "优化idp_ref"
  Constant7/1 -> Sum3/1
  Gain12/1 -> Sum3/2
  Ramp4/1 -> Saturation1/1, Saturation3/1, Saturation2/1, Saturation4/1
  Saturation4/1 -> Gain12/1  "斜坡"
  Saturation1/1 -> Gain14/1  "斜坡"
  Gain14/1 -> Goto8/1
  Gain5/1 -> Goto9/1  "idn_ref"
  Saturation3/1 -> Gain9/1
  MATLAB Function5/1(y) -> [wt]
  [I1d_p] -> dq轴功率计算/5(id_p)
  [I1q_p] -> dq轴功率计算/6(iq_p)
  [I1d_n] -> dq轴功率计算/7(id_n)
  [I1q_n] -> dq轴功率计算/8(iq_n)
  dq轴功率计算/1(P1) -> Mux/1
  dq轴功率计算/2(Q1) -> Mux/2
  Mux/1 -> Scope5/1, Display/1
  IBR1输出电流正负序分离1/1(d+) -> [vd_p]
  IBR1输出电流正负序分离1/2(q+) -> [vq_p]
  IBR1输出电流正负序分离1/3(d-) -> [vd_n]
  IBR1输出电流正负序分离1/4(q-) -> [vq_n]
  [vd_p] -> dq轴功率计算/1(vd_p)
  [vq_p] -> dq轴功率计算/2(vq_p)
  [vd_n] -> dq轴功率计算/3(vd_n)
  [vq_n] -> dq轴功率计算/4(vq_n)
  [vd_n] -> IBR1/3(vcd_n)
  [vq_n] -> IBR1/4(vcq_n)
  [vq_p] -> IBR1/2(vcq_p)
  [vd_p] -> IBR1/1(vcd_p)
  IBR1/2(Vc_n) -> Scope6/2
  IBR1/1(Vc_p) -> Scope6/1
  IBR1/3(VUF) -> Scope6/3
  connections:
  Bus 1/RConn3 -- Conn3/RConn1
  Bus 1/RConn2 -- Conn2/RConn1
  Bus 1/RConn1 -- Conn1/RConn1
  Controlled Voltage Source2/LConn1 -- Controlled Voltage Source/LConn1 -- Controlled Voltage Source1/LConn1
  Controlled Voltage Source/RConn1 -- Series RLC Branch3/LConn1
  Controlled Voltage Source2/RConn1 -- Series RLC Branch4/LConn1
  Controlled Voltage Source1/RConn1 -- Series RLC Branch5/LConn1
  Series RLC Branch4/RConn1 -- Series RLC Branch10/LConn1 -- Series RLC Branch7/LConn1
  Series RLC Branch7/RConn1 -- Bus 1/LConn2
  Bus 1/LConn1 -- Series RLC Branch6/RConn1
  Series RLC Branch6/LConn1 -- Series RLC Branch3/RConn1 -- Series RLC Branch9/LConn1
  Series RLC Branch5/RConn1 -- Series RLC Branch11/LConn1 -- Series RLC Branch8/LConn1
  Series RLC Branch8/RConn1 -- Bus 1/LConn3
  Ground/LConn1 -- Series RLC Branch11/RConn1 -- Series RLC Branch9/RConn1 -- Series RLC Branch10/RConn1

== system Main_Model/Unbalance/Grid/negative_sequence_dq>>abc4 ==
  note: alpha_beta_0
  note: 0
  note: q
  note: d
  dq0 : Inport
  theta : Inport  Port=2
  Demux3 : Demux  Outputs=3
      settings: DisplayOption=none
  MATLAB Function : MATLAB Function  TreatAsAtomicUnit=on
  Mux1 : Mux  Inputs=3
  dq0>>alpha_beta_0 : Subsystem
  abc : Outport
  wires:
  theta/1 -> MATLAB Function/3(theta)
  Demux3/3 -> Mux1/3
  MATLAB Function/2(beta) -> Mux1/2
  MATLAB Function/1(alpha) -> Mux1/1
  Demux3/2 -> MATLAB Function/2(q)
  Demux3/1 -> MATLAB Function/1(d)
  dq0>>alpha_beta_0/1(abc) -> abc/1
  Mux1/1 -> dq0>>alpha_beta_0/1(alpha_beta_0)
  dq0/1 -> Demux3/1

== system Main_Model/Unbalance/Grid/positive_sequence_dq>>abc1 ==
  note: alpha axis 与A axis 重合
  note: alpha_beta_0
  note: 0
  note: q
  note: d
  dq0 : Inport
  theta : Inport  Port=2
  Demux3 : Demux  Outputs=3
      settings: DisplayOption=none
  MATLAB Function : MATLAB Function  TreatAsAtomicUnit=on
  Mux1 : Mux  Inputs=3
  dq0>>alpha_beta_0 : Subsystem
  abc : Outport
  wires:
  theta/1 -> MATLAB Function/3(theta)
  Demux3/3 -> Mux1/3
  MATLAB Function/2(beta) -> Mux1/2
  MATLAB Function/1(alpha) -> Mux1/1
  Demux3/2 -> MATLAB Function/2(q)
  Demux3/1 -> MATLAB Function/1(d)
  dq0>>alpha_beta_0/1(abc) -> abc/1
  Mux1/1 -> dq0>>alpha_beta_0/1(alpha_beta_0)
  dq0/1 -> Demux3/1
